simulink model "robot_capteur_etu"  (R2021b)
settings: Solver=VariableStepAuto  StartTime=0.0  StopTime=10.0  RelTol=1e-3
values from neighbouring files (symbols this model uses):
  K = -place(A,B,V)    [matrices.m]    (also in simu_robot_etu.m = [0.6700  19.9055   1.0747   1.9614])
  t0 = 0    [simu_robot_etu.m]
  ue = 0    [simu_robot_etu.m]
  x0 = [0 pi/10 0 0]    [simu_robot_etu.m]
  xe = [0 0 0 0]'    [simu_robot_etu.m]
settings Model: Creator=roussake  LastModifiedBy=roussake

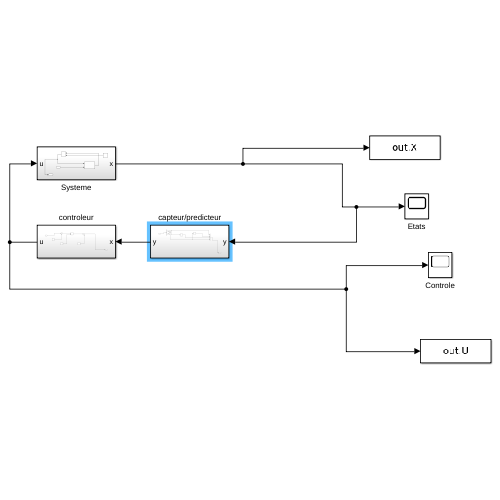
[thumbnail: Simulink's stored preview of the top-level diagram]
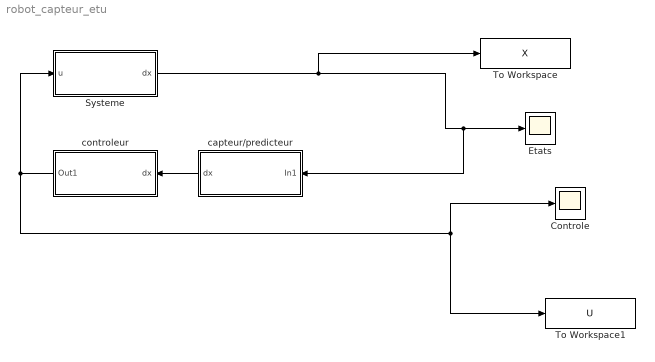
== system robot_capteur_etu ==
  Controle : Scope
  Etats : Scope
  Systeme : Subsystem
  To Workspace : ToWorkspace  VariableName=X  SaveFormat=Timeseries  SampleTime=-1
  To Workspace1 : ToWorkspace  VariableName=U  SaveFormat=Timeseries  SampleTime=-1
  capteur/predicteur : Subsystem
  controleur : Subsystem
  wires:
  Systeme/1(dx) -> capteur/predicteur/1(In1), Etats/1, To Workspace/1
  controleur/1(Out1) -> Systeme/1(u), Controle/1, To Workspace1/1
  capteur/predicteur/1(dx) -> controleur/1(dx)

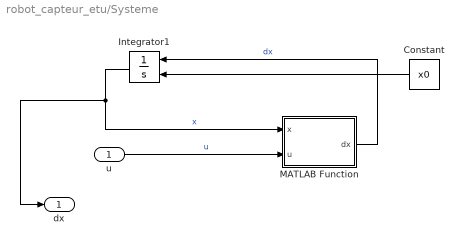
== system robot_capteur_etu/Systeme ==
  u : Inport
  Constant : Constant  Value=x0
  Integrator1 : Integrator  InitialConditionSource=external  InitialCondition=t0
  MATLAB Function : MATLAB Function  TreatAsAtomicUnit=on
  dx : Outport
  wires:
  MATLAB Function/1(dx) -> Integrator1/1  "dx"
  Constant/1 -> Integrator1/2
  u/1 -> MATLAB Function/2(u)  "u"
  Integrator1/1 -> dx/1, MATLAB Function/1(x)  "x"

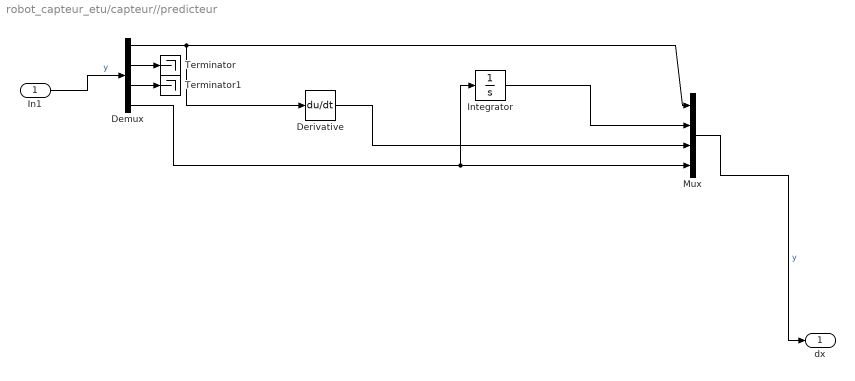
== system robot_capteur_etu/capteur//predicteur ==
  In1 : Inport
  Demux : Demux
  Derivative : Derivative
  Integrator : Integrator
  Mux : Mux
  Terminator : Terminator
  Terminator1 : Terminator
  dx : Outport
  wires:
  In1/1 -> Demux/1  "y"
  Mux/1 -> dx/1  "y"
  Demux/1 -> Derivative/1, Mux/1
  Derivative/1 -> Mux/3
  Demux/4 -> Integrator/1, Mux/4
  Integrator/1 -> Mux/2
  Demux/2 -> Terminator/1
  Demux/3 -> Terminator1/1

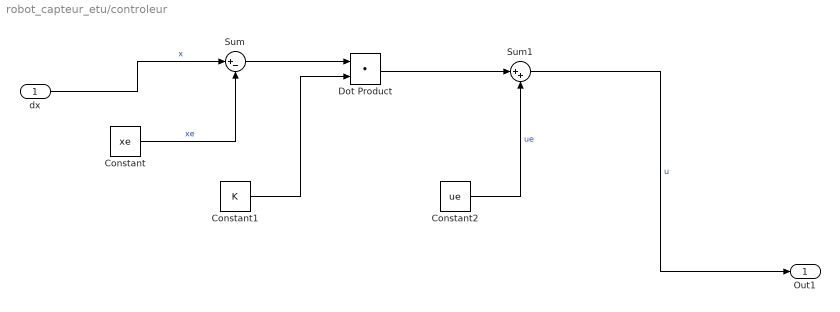
== system robot_capteur_etu/controleur ==
  dx : Inport
  Constant : Constant  Value=xe
  Constant1 : Constant  Value=K
  Constant2 : Constant  Value=ue
  Dot Product : DotProduct  InputSameDT=on  OutDataTypeStr=Inherit: Inherit via internal rule
  Sum : Sum  Inputs=|+-
  Sum1 : Sum  Inputs=|++
  Out1 : Outport
  wires:
  dx/1 -> Sum/1  "x"
  Constant/1 -> Sum/2  "xe"
  Sum/1 -> Dot Product/1
  Dot Product/1 -> Sum1/1
  Constant2/1 -> Sum1/2  "ue"
  Sum1/1 -> Out1/1  "u"
  Constant1/1 -> Dot Product/2

== matlab function robot_capteur_etu/Systeme/MATLAB Function ==
  data: x input; u input; dx output
function dx   = fonction( x, u)
%   Dynamic equations of motion of the segway on an axis.
%   Inputs: - x = [theta psi dtheta dpsi]
%               theta: average angle of the wheels      [rad]
%               psi: body pitch angle                   [rad]
%               dtheta: average velocity of the wheels  [rad/s]
%               dpsi: body pitch velocity               [rad/s]
%          - u: DC motor voltage (same value for both motors) [V]

    % State
    psi = x(2);
    dtheta = x(3);
    dpsi = x(4);

    % Parameters
    
    g = 9.81;           % gravity acceleration [m/sec^2]
    m = 0.03;           % wheel weight [kg]
    R = 0.04;           % wheel radius [m]
    Jw = m*R^2/2;       % wheel inertia moment [kg*m^2]
    M = 0.6;            % body weight [kg]
    H = 0.144;          % body height [m]
    L = H/2;            % distance of the center of mass from the wheel axle [m]
    Jpsi = M*L^2/3;     % body pitch inertia [kgm^2]
    Jm = 1e-5;          % DC motor inertia moment [kgm^2]
    Rm = 6.69;          % DC motor resistance [Ohm]
    Kb = 0.468;         % DC motor back EMF constant [Vsec/rad]
    Kt = 0.317;         % DC motor torque constant [Nm/A]
    n = 1;              % gear ratio
    fm = 0.0022;        % friction coefficient between body and DC motor
    fw = 0;             % friction coefficient between wheel and floor
    
    % Equations of motion
    c1 = (2*m+M)*R^2 + 2*Jw + 2*n^2*Jm;
    c2 = M*L*R*cos(psi) - 2*n^2*Jm;
    c3 = -M*L*R*dpsi^2*sin(psi);
    c4 = M*L^2 + Jpsi + 2*n^2*Jm;
    c5 = -M*g*L*sin(psi);

    alpha = Kt/Rm;
    beta = Kt*Kb/Rm + fm;

    Ftheta = alpha*(2*u) - 2*(beta+fw)*dtheta + 2*beta*dpsi;
    Fpsi = -alpha*(2*u) + 2*beta*dtheta - 2*beta*dpsi;

    ddtheta = (c4*c3 - c2*c5 + c4*Ftheta - c2*Fpsi)/(c4*c1 - c2^2);
    ddpsi = (Fpsi- c2*ddtheta - c5)/c4;
    dx = [dtheta dpsi ddtheta ddpsi]';

end
